simulink subsystem "ECI2GroundTrack"  (R2021a)
settings: Solver=VariableStepAuto  StartTime=0.0  StopTime=10.0  RelTol=1e-3
undefined symbols (not defined in the file): IAU
libraries: aerolibtransform2 x1
settings Model: Creator=Laura  LastModifiedBy=Laura

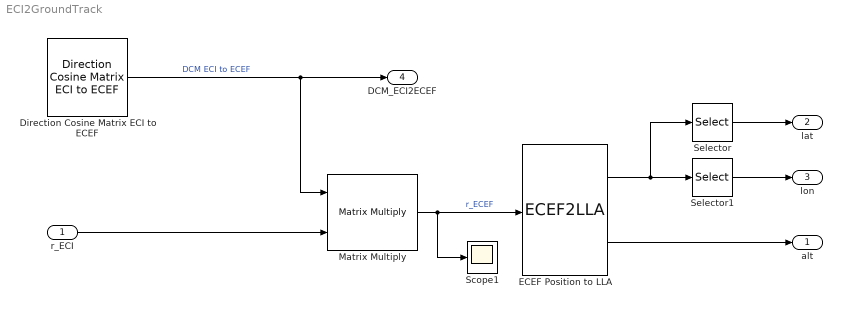
== system ECI2GroundTrack ==
  r_ECI : Inport
  Direction Cosine Matrix ECI to ECEF : aerolibtransform2/Direction Cosine Matrix ECI to ECEF  red=IAU-2000/2006  year=year  month=February  day=1  hour=hour  min=min  sec=sec  deltaT=None  errorflag=Error  extraparamflag=off
      settings: AttributesFormatString=%<red>  SourceProductBaseCode=AE
  ECEF Position to LLA : ECEF2LLA
  Matrix Multiply : Product  Multiplication=Matrix(*)
  Scope1 : Scope
  Selector : Selector  InputPortWidth=2  IndexOptions=Index vector (dialog)  Indices=[1]  OutputSizes=1
  Selector1 : Selector  InputPortWidth=2  IndexOptions=Index vector (dialog)  Indices=[2]  OutputSizes=1
  alt : Outport
  lat : Outport  Port=2
  lon : Outport  Port=3
  DCM_ECI2ECEF : Outport  Port=4
  wires:
  Matrix Multiply/1 -> Scope1/1, ECEF Position to LLA/1  "r_ECEF"
  r_ECI/1 -> Matrix Multiply/2
  ECEF Position to LLA/2 -> alt/1
  Direction Cosine Matrix ECI to ECEF/1 -> DCM_ECI2ECEF/1, Matrix Multiply/1  "DCM ECI to ECEF"
  ECEF Position to LLA/1 -> Selector/1, Selector1/1
  Selector/1 -> lat/1
  Selector1/1 -> lon/1
